simulink library "lib_signals_to_nByteLayout_withCrc"  (R2020a)
settings: Solver=VariableStepAuto  StartTime=0.0  StopTime=10.0  RelTol=1e-3
settings Model: Creator=Administrator  LastModifiedBy=Administrator
settings DataIOCC: ReturnWorkspaceOutputs=off
settings DebuggingCC: ArithmeticOperatorsInVariantConditions=warning
settings SFSimCC: SimUseLocalCustomCode=off  CustomCodeUndefinedFunction=UseInterfaceOnly
settings RTWCC: RTWUseLocalCustomCode=off

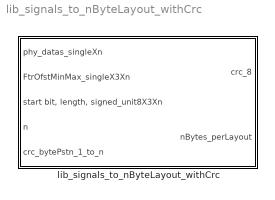
== system lib_signals_to_nByteLayout_withCrc ==
  lib_signals_to_nByteLayout_withCrc : Subsystem

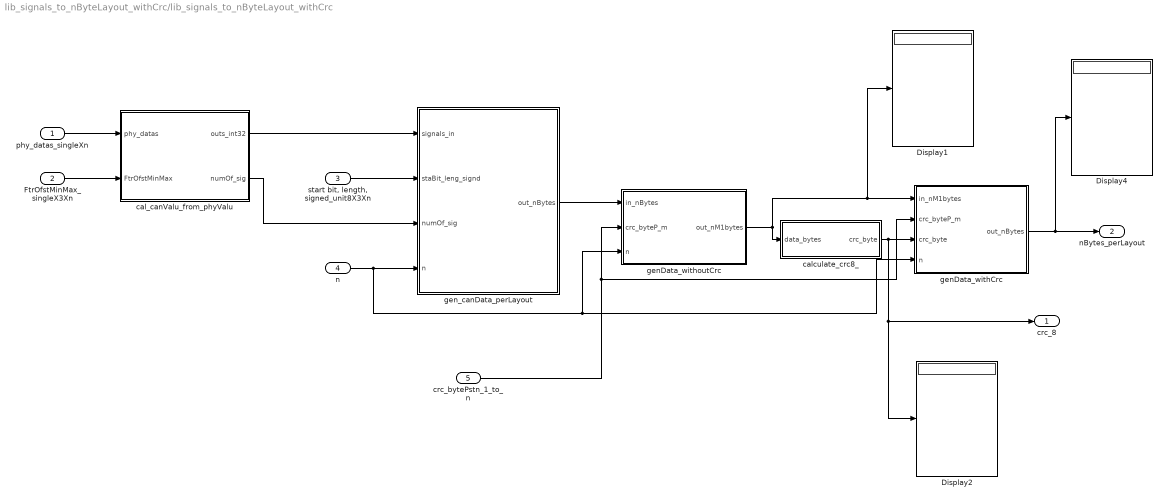
== system lib_signals_to_nByteLayout_withCrc/lib_signals_to_nByteLayout_withCrc ==
  phy_datas_singleXn : Inport  OutDataTypeStr=single
  FtrOfstMinMax_singleX3Xn : Inport  Port=2  OutDataTypeStr=single
  "start bit, length, signed_unit8X3Xn" : Inport  Port=3  OutDataTypeStr=uint8
  n : Inport  Port=4  OutDataTypeStr=uint8  PortDimensions=1
  crc_bytePstn_1_to_n : Inport  Port=5  OutDataTypeStr=uint8  PortDimensions=1
  Display1 : Display
  Display2 : Display
  Display4 : Display
  cal_canValu_from_phyValu : MATLAB Function  TreatAsAtomicUnit=on
  calculate_crc8_ : MATLAB Function  TreatAsAtomicUnit=on
  genData_withCrc : MATLAB Function  TreatAsAtomicUnit=on
  genData_withoutCrc : MATLAB Function  TreatAsAtomicUnit=on
  gen_canData_perLayout : MATLAB Function  TreatAsAtomicUnit=on
  crc_8 : Outport  OutDataTypeStr=uint8  PortDimensions=1  VectorParamsAs1DForOutWhenUnconnected=off
  nBytes_perLayout : Outport  Port=2  OutDataTypeStr=uint8  VectorParamsAs1DForOutWhenUnconnected=off
  wires:
  cal_canValu_from_phyValu/2(numOf_sig) -> gen_canData_perLayout/3(numOf_sig)
  calculate_crc8_/1(crc_byte) -> crc_8/1, Display2/1, genData_withCrc/3(crc_byte)
  FtrOfstMinMax_singleX3Xn/1 -> cal_canValu_from_phyValu/2(FtrOfstMinMax)
  genData_withCrc/1(out_nBytes) -> nBytes_perLayout/1, Display4/1
  "start bit, length, signed_unit8X3Xn"/1 -> gen_canData_perLayout/2(staBit_leng_signd)
  genData_withoutCrc/1(out_nM1bytes) -> genData_withCrc/1(in_nM1bytes), Display1/1, calculate_crc8_/1(data_bytes)
  crc_bytePstn_1_to_n/1 -> genData_withoutCrc/2(crc_byteP_m), genData_withCrc/2(crc_byteP_m)
  gen_canData_perLayout/1(out_nBytes) -> genData_withoutCrc/1(in_nBytes)
  cal_canValu_from_phyValu/1(outs_int32) -> gen_canData_perLayout/1(signals_in)
  phy_datas_singleXn/1 -> cal_canValu_from_phyValu/1(phy_datas)
  n/1 -> genData_withoutCrc/3(n), genData_withCrc/4(n), gen_canData_perLayout/4(n)

== matlab function lib_signals_to_nByteLayout_withCrc/calculate_crc8_ ==
  data: data_bytes input uint8 size=8; crc_byte output uint8 size=1
% function crc8 = fcn(byte_data, bytes)
function crc_byte = fcn(data_bytes)


    t_crc = uint8(hex2dec('ff'));
    [bytes, temp] = size( data_bytes );
    
    for f = 1:bytes
        t_crc = bitxor(data_bytes(f),t_crc);

        for b = 1:8

             if(bitand( t_crc,hex2dec('80') ) ~= 0)  
                   t_crc = bitshift( t_crc,1 );
                   t_crc = bitxor( t_crc,hex2dec('1d') );

             else
                   t_crc = bitshift(t_crc,1);

             end
        end
    end

    %equivalent of c coding: ~t_crc
    crc_byte = bitxor(t_crc, hex2dec('ff'));

== matlab function lib_signals_to_nByteLayout_withCrc/gen_canData_perLayout ==
  data staBit_leng_signd settings: description=start bit, length, signed
  data: signals_in input int32; out_nBytes output uint8 size=8; staBit_leng_signd input uint8; numOf_sig input uint8 size=1; n input uint8 size=1
function out_nBytes = fcn(signals_in, staBit_leng_signd, numOf_sig, n)

out_nBytes = zeros(n, 1, 'uint8');

for sig = 1 : numOf_sig 
    % get data
    data = signals_in(sig);
    strBit =  staBit_leng_signd( (sig-1)*3 + 1 ) + 1; % +1 is because we use matlab counting inside this function
    leng   =  staBit_leng_signd( (sig-1)*3 + 2 );
    signed  =  staBit_leng_signd( (sig-1)*3 + 3 );
    
    
    % determine the address (row/byte and column/bit) of the starting bit
%    row_byt = uint8(floor(strBit/uint8(8) ) );
    row_byt = uint8( floor( single(strBit-1)/single(8) ) ) + 1;   % -1 is to start from 0 instead of 1 
%    col_bit = strBit - (row_byt - 1) * 8; 
    col_bit = mod(strBit-1, 8) + 1;   % -1 is to start from 0 instead of 1
    
    % copy each bit in data into the CAN layout
    for data_b = 1 :1 :leng
      
        if signed && (data_b == leng)    % special case for signed input and at the msb
            v = bitget(data, 32 );        % msb of the input data int32                    
        else    % all regular case
            v = bitget( data, data_b );     
        end
        
        out_nBytes(row_byt) = bitset( out_nBytes(row_byt), col_bit, v);
        
        col_bit = col_bit + 1;
        if (col_bit > 8)
            col_bit = uint8(1);
            row_byt = row_byt - 1;   % this is the way layout goes
            
        end
    end
    
    
end

== matlab function lib_signals_to_nByteLayout_withCrc/genData_withCrc ==
  data crc_byteP_m settings: description=start bit, length, signed
  data crc_byte settings: description=start bit, length, signed
  data: in_nM1bytes input uint8; crc_byteP_m input uint8 size=1; out_nBytes output uint8 size=8; crc_byte input uint8 size=1; n input uint8 size=1
function out_nBytes  = fcn(in_nM1bytes, crc_byteP_m, crc_byte, n)

out_nBytes = zeros(n, 1, 'uint8');
in_pstn  = uint8(1);
out_pstn = uint8(1);

while out_pstn <= n   
    if out_pstn == crc_byteP_m
        out_nBytes(out_pstn) = crc_byte;   
    else
        out_nBytes(out_pstn) = in_nM1bytes(in_pstn);       
        in_pstn = in_pstn + 1;
    end
    out_pstn = out_pstn + 1;
end

== matlab function lib_signals_to_nByteLayout_withCrc/genData_withoutCrc ==
  data crc_byteP_m settings: description=start bit, length, signed
  data: in_nBytes input uint8; crc_byteP_m input uint8 size=1; out_nM1bytes output uint8 size=8; n input uint8 size=1
function out_nM1bytes  = fcn(in_nBytes, crc_byteP_m, n)

out_nM1bytes = zeros(n-1,1, 'uint8');

byte_in  = uint8(1);
byte_out = uint8(1);

while byte_in <= n   
    if byte_in == crc_byteP_m
        
    else
        out_nM1bytes(byte_out) = in_nBytes(byte_in);       
        byte_out = byte_out + 1;
    end
    byte_in = byte_in + 1;
end

== matlab function lib_signals_to_nByteLayout_withCrc/cal_canValu_from_phyValu ==
  data FtrOfstMinMax settings: description=factor, offset, min, max
  data: outs_int32 output int32 size=100; phy_datas input single; FtrOfstMinMax input single; numOf_sig output uint8 size=1
function [outs_int32,numOf_sig] = fcn(phy_datas, FtrOfstMinMax)



temp = size(phy_datas);
numOf_sig = uint8(temp(1));

outs_int32 = zeros(numOf_sig, 1, 'int32');

for sig = 1 : numOf_sig 
    in_single = phy_datas(sig);
    i_base = (sig-1) * 4 ;
    factor = FtrOfstMinMax( i_base + 1);
    offset = FtrOfstMinMax( i_base + 2);
    min_v  = FtrOfstMinMax( i_base + 3);
    max_v  = FtrOfstMinMax( i_base + 4);
    
    if (in_single < min_v ) || (in_single > max_v )
        "Error 1319"
    end
    out_int32       = int32( (in_single - offset)/factor );    
    outs_int32(sig) = out_int32;
end
